simulink model "rou1_huibao_orthotropic_control"  (R2019b)
settings: Solver=ode23t  StartTime=0.0  StopTime=20  RelTol=1e-3
values from neighbouring files (symbols this model uses):
  I1 = 1    [HRGinitial.m]    (also in hrg_constr.m; untitled.m = 2000)
  I2 = 2500    [HRGinitial.m]    (also in hrg_constr.m; untitled.m = 1)
  I3 = 2000    [HRGinitial.m]    (also in hrg_constr.m = 2500; untitled.m = 2500)
  I4 = 2500    [HRGinitial.m]    (also in hrg_constr.m = 2000; untitled.m)
  K = 1.122    [HRGinitial.m]
  P1 = 0.2    [HRGinitial.m]    (also in hrg_constr.m; untitled.m = 40)
  P2 = 35    [HRGinitial.m]    (also in hrg_constr.m; untitled.m = 0.2)
  P3 = 40    [HRGinitial.m]    (also in hrg_constr.m = 35; untitled.m = 35)
  P4 = 35    [HRGinitial.m]    (also in hrg_constr.m = 40; untitled.m)
  x0 = [a*cos(omega*t+phi0)*cos(2*theta)-q*sin(omega*t+phi0)*sin(2*theta) ... (first row only)    [HRGinitial.m]
libraries: simulink x11, dsparch4 x4, dspswit3 x1, eeSinusoidalMeasurement x1, eeGeneralControl x1
settings Model: Creator=Administrator  LastModifiedBy=Administrator
settings SolverCC: AlgebraicLoopSolver=LineSearch

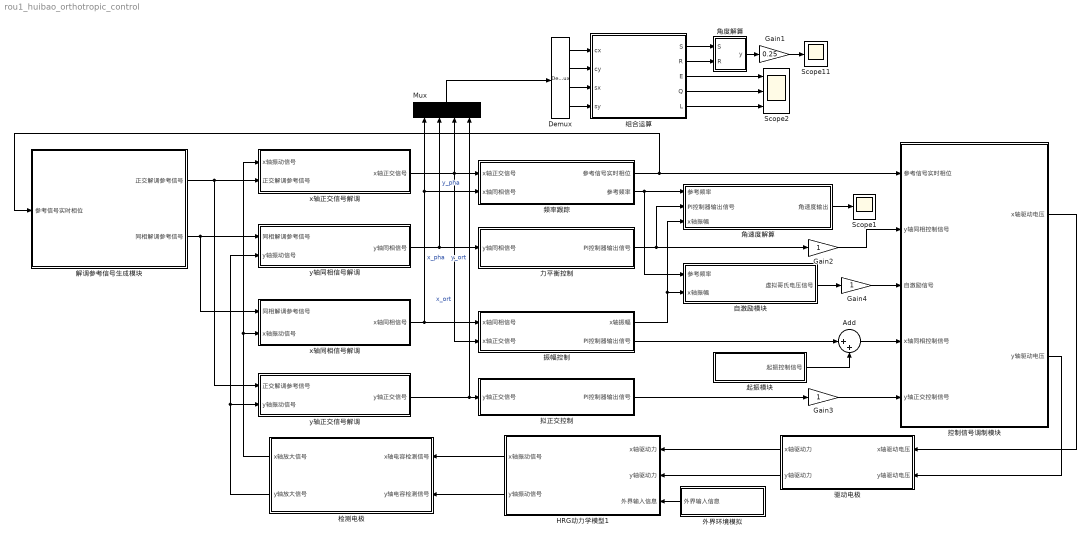
== system rou1_huibao_orthotropic_control ==
  Add : Sum  Inputs=|++
  Demux : Demux
  Gain1 : Gain  Gain=0.25
  Gain2 : Gain
  Gain3 : Gain
  Gain4 : Gain
  HRG动力学模型1 : Subsystem
  Mux : Mux
  Scope1 : Scope
  Scope11 : Scope
  Scope2 : Scope  NumInputPorts=3
  x轴同相信号解调 : Subsystem
  x轴正交信号解调 : Subsystem
  y轴同相信号解调 : Subsystem
  y轴正交信号解调 : Subsystem
  力平衡控制 : Subsystem
  外界环境模拟 : Subsystem
  拟正交控制 : Subsystem
  振幅控制 : Subsystem
  控制信号调制模块 : Subsystem
  检测电极 : Subsystem
  组合运算 : MATLAB Function  TreatAsAtomicUnit=on
  自激励模块 : Subsystem
  角度解算 : MATLAB Function  TreatAsAtomicUnit=on
  角速度解算 : Subsystem
  解调参考信号生成模块 : Subsystem
  起振模块 : Subsystem
  频率跟踪 : Subsystem
  驱动电极 : Subsystem
  wires:
  驱动电极/2(y轴驱动力) -> HRG动力学模型1/2(y轴驱动力)
  驱动电极/1(x轴驱动力) -> HRG动力学模型1/1(x轴驱动力)
  HRG动力学模型1/1(x轴振动信号) -> 检测电极/1(x轴电容检测信号)
  HRG动力学模型1/2(y轴振动信号) -> 检测电极/2(y轴电容检测信号)
  外界环境模拟/1(外界输入信息) -> HRG动力学模型1/3(外界输入信息)
  Demux/2 -> 组合运算/2(cy)
  组合运算/5(L) -> Scope2/3
  组合运算/3(E) -> Scope2/1
  解调参考信号生成模块/2(同相解调参考信号) -> y轴同相信号解调/1(同相解调参考信号), x轴同相信号解调/1(同相解调参考信号)
  Demux/3 -> 组合运算/3(sx)
  组合运算/2(R) -> 角度解算/2(R)
  自激励模块/1(虚拟哥氏电压信号) -> Gain4/1
  x轴同相信号解调/1(x轴同相信号) -> 振幅控制/1(x轴同相信号), 频率跟踪/2(x轴同相信号), Mux/1  "x_pha"
  Mux/1 -> Demux/1
  y轴同相信号解调/1(y轴同相信号) -> 力平衡控制/1(y轴同相信号), Mux/2  "y_pha"
  检测电极/2(y轴放大信号) -> y轴同相信号解调/2(y轴振动信号), y轴正交信号解调/2(y轴振动信号)
  控制信号调制模块/2(y轴驱动电压) -> 驱动电极/2(y轴驱动电压)
  组合运算/1(S) -> 角度解算/1(S)
  Gain1/1 -> Scope11/1
  检测电极/1(x轴放大信号) -> x轴正交信号解调/1(x轴振动信号), x轴同相信号解调/2(x轴振动信号)
  Add/1 -> 控制信号调制模块/4(x轴同相控制信号)
  振幅控制/1(x轴振幅) -> 角速度解算/3(x轴振幅), 自激励模块/2(x轴振幅)
  解调参考信号生成模块/1(正交解调参考信号) -> x轴正交信号解调/2(正交解调参考信号), y轴正交信号解调/1(正交解调参考信号)
  y轴正交信号解调/1(y轴正交信号) -> 拟正交控制/1(y轴正交信号), Mux/4  "y_ort"
  x轴正交信号解调/1(x轴正交信号) -> Mux/3, 频率跟踪/1(x轴正交信号), 振幅控制/2(x轴正交信号)  "x_ort"
  角速度解算/1(角速度输出) -> Scope1/1
  角度解算/1(y) -> Gain1/1
  组合运算/4(Q) -> Scope2/2
  频率跟踪/1(参考信号实时相位) -> 控制信号调制模块/1(参考信号实时相位), 解调参考信号生成模块/1(参考信号实时相位)
  控制信号调制模块/1(x轴驱动电压) -> 驱动电极/1(x轴驱动电压)
  起振模块/1(起振控制信号) -> Add/2
  力平衡控制/1(PI控制器输出信号) -> 角速度解算/2(PI控制器输出信号), Gain2/1
  Demux/1 -> 组合运算/1(cx)
  振幅控制/2(PI控制器输出信号) -> Add/1
  Demux/4 -> 组合运算/4(sy)
  频率跟踪/2(参考频率) -> 角速度解算/1(参考频率), 自激励模块/1(参考频率)
  拟正交控制/1(PI控制器输出信号) -> Gain3/1
  Gain2/1 -> 控制信号调制模块/2(y轴同相控制信号)
  Gain3/1 -> 控制信号调制模块/5(y轴正交控制信号)
  Gain4/1 -> 控制信号调制模块/3(自激励信号)

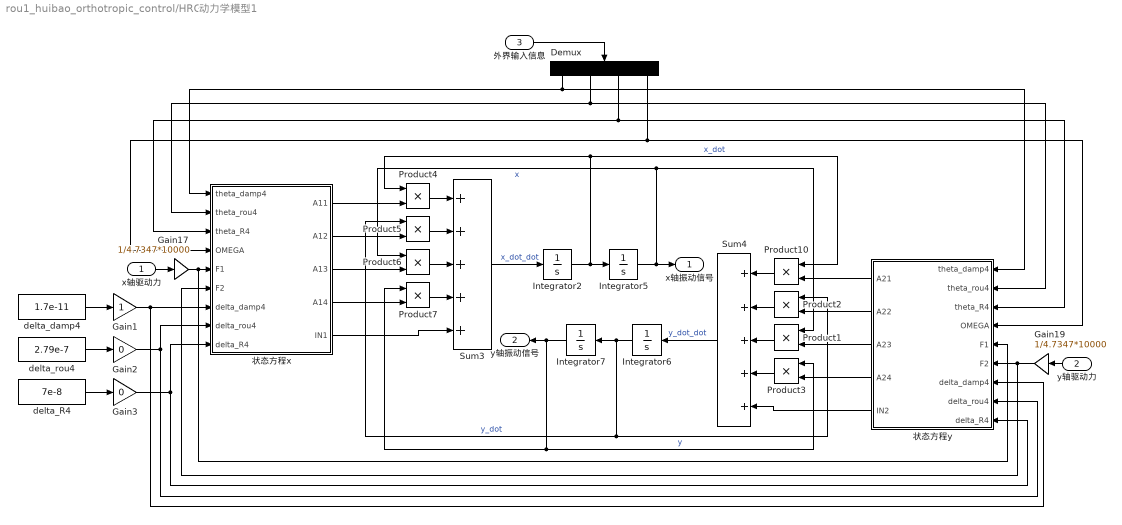
== system rou1_huibao_orthotropic_control/HRG动力学模型1 ==
  x轴驱动力 : Inport
  y轴驱动力 : Inport  Port=2
  外界输入信息 : Inport  Port=3
  Demux : Demux
  Gain1 : Gain
  Gain17 : Gain  Gain=1/4.7347*10000
  Gain19 : Gain  Gain=1/4.7347*10000
  Gain2 : Gain  Gain=0
  Gain3 : Gain  Gain=0
  Integrator2 : Integrator  InitialCondition=x0(3)
  Integrator5 : Integrator  InitialCondition=x0(1)
  Integrator6 : Integrator  InitialCondition=x0(4)
  Integrator7 : Integrator  InitialCondition=x0(2)
  Product{1..7,10} (8 alike) : Product
  Sum3 : Sum  Inputs=+++++
  Sum4 : Sum  Inputs=+++++
  delta_R4 : Constant  Value=7e-8
  delta_damp4 : Constant  Value=1.7e-11
  delta_rou4 : Constant  Value=2.79e-7
  状态方程x : MATLAB Function  TreatAsAtomicUnit=on
  状态方程y : MATLAB Function  TreatAsAtomicUnit=on
  x轴振动信号 : Outport
  y轴振动信号 : Outport  Port=2
  wires:
  y轴驱动力/1 -> Gain19/1
  x轴驱动力/1 -> Gain17/1
  Integrator2/1 -> Product4/1, Product10/1, Integrator5/1  "x_dot"
  Integrator6/1 -> Product2/1, Product5/1, Integrator7/1  "y_dot"
  Integrator7/1 -> Product3/1, Product7/1, y轴振动信号/1  "y"
  Sum3/1 -> Integrator2/1  "x_dot_dot"
  Integrator5/1 -> Product6/1, Product1/1, x轴振动信号/1  "x"
  Sum4/1 -> Integrator6/1  "y_dot_dot"
  状态方程x/5(IN1) -> Sum3/5
  Gain17/1 -> 状态方程y/5(F1), 状态方程x/5(F1)
  Gain19/1 -> 状态方程y/6(F2), 状态方程x/6(F2)
  Demux/1 -> 状态方程x/1(theta_damp4), 状态方程y/1(theta_damp4)
  Demux/2 -> 状态方程x/2(theta_rou4), 状态方程y/2(theta_rou4)
  Demux/3 -> 状态方程x/3(theta_R4), 状态方程y/3(theta_R4)
  Demux/4 -> 状态方程x/4(OMEGA), 状态方程y/4(OMEGA)
  外界输入信息/1 -> Demux/1
  状态方程y/5(IN2) -> Sum4/5
  Product1/1 -> Sum4/3
  Product2/1 -> Sum4/2
  Product10/1 -> Sum4/1
  Product3/1 -> Sum4/4
  Product4/1 -> Sum3/1
  Product5/1 -> Sum3/2
  Product6/1 -> Sum3/3
  Product7/1 -> Sum3/4
  状态方程x/1(A11) -> Product4/2
  状态方程x/2(A12) -> Product5/2
  状态方程x/3(A13) -> Product6/2
  状态方程x/4(A14) -> Product7/2
  状态方程y/1(A21) -> Product10/2
  状态方程y/2(A22) -> Product2/2
  状态方程y/3(A23) -> Product1/2
  状态方程y/4(A24) -> Product3/2
  delta_damp4/1 -> Gain1/1
  delta_R4/1 -> Gain3/1
  Gain1/1 -> 状态方程y/7(delta_damp4), 状态方程x/7(delta_damp4)
  delta_rou4/1 -> Gain2/1
  Gain2/1 -> 状态方程x/8(delta_rou4), 状态方程y/8(delta_rou4)
  Gain3/1 -> 状态方程y/9(delta_R4), 状态方程x/9(delta_R4)

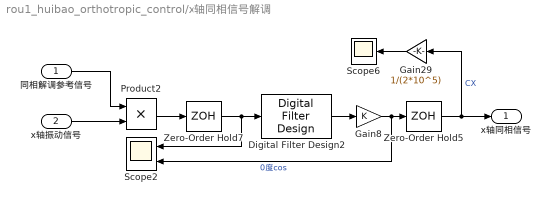
== system rou1_huibao_orthotropic_control/x轴同相信号解调 ==
  同相解调参考信号 : Inport
  x轴振动信号 : Inport  Port=2
  Digital Filter Design2 : dsparch4/Digital Filter Design  mwdsp_browser_bugfix_var=off
  Gain29 : Gain  Gain=1/(2*10^5)
  Gain8 : Gain  Gain=K
  Product2 : Product
  Scope2 : Scope  NumInputPorts=2
  Scope6 : Scope
  Zero-Order Hold5 : ZeroOrderHold  SampleTime=1/1000
  Zero-Order Hold7 : ZeroOrderHold  SampleTime=1/125000
  x轴同相信号 : Outport
  wires:
  Zero-Order Hold7/1 -> Scope2/1, Digital Filter Design2/1
  Zero-Order Hold5/1 -> Gain29/1, x轴同相信号/1  "CX"
  Product2/1 -> Zero-Order Hold7/1
  同相解调参考信号/1 -> Product2/1
  Gain8/1 -> Scope2/2, Zero-Order Hold5/1  "0度cos"
  Digital Filter Design2/1 -> Gain8/1
  x轴振动信号/1 -> Product2/2
  Gain29/1 -> Scope6/1

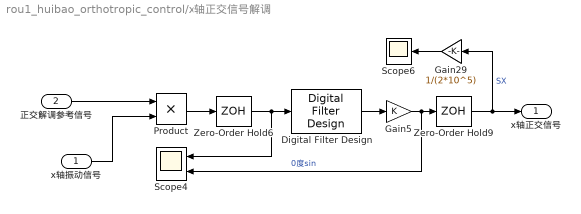
== system rou1_huibao_orthotropic_control/x轴正交信号解调 ==
  x轴振动信号 : Inport
  正交解调参考信号 : Inport  Port=2
  Digital Filter Design : dsparch4/Digital Filter Design  mwdsp_browser_bugfix_var=off
  Gain29 : Gain  Gain=1/(2*10^5)
  Gain5 : Gain  Gain=K
  Product : Product
  Scope4 : Scope  NumInputPorts=2
  Scope6 : Scope
  Zero-Order Hold6 : ZeroOrderHold  SampleTime=1/125000
  Zero-Order Hold9 : ZeroOrderHold  SampleTime=1/1000
  x轴正交信号 : Outport
  wires:
  Product/1 -> Zero-Order Hold6/1
  Zero-Order Hold9/1 -> Gain29/1, x轴正交信号/1  "SX"
  Gain5/1 -> Scope4/2, Zero-Order Hold9/1  "0度sin"
  Zero-Order Hold6/1 -> Scope4/1, Digital Filter Design/1
  x轴振动信号/1 -> Product/2
  Digital Filter Design/1 -> Gain5/1
  正交解调参考信号/1 -> Product/1
  Gain29/1 -> Scope6/1

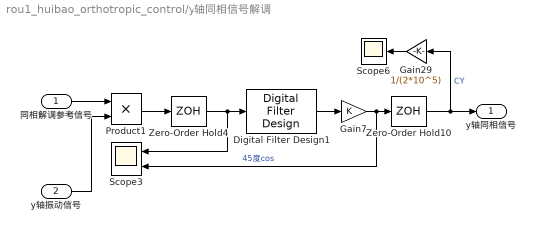
== system rou1_huibao_orthotropic_control/y轴同相信号解调 ==
  同相解调参考信号 : Inport
  y轴振动信号 : Inport  Port=2
  Digital Filter Design1 : dsparch4/Digital Filter Design  mwdsp_browser_bugfix_var=off
  Gain29 : Gain  Gain=1/(2*10^5)
  Gain7 : Gain  Gain=K
  Product1 : Product
  Scope3 : Scope  NumInputPorts=2
  Scope6 : Scope
  Zero-Order Hold10 : ZeroOrderHold  SampleTime=1/1000
  Zero-Order Hold4 : ZeroOrderHold  SampleTime=1/125000
  y轴同相信号 : Outport
  wires:
  Gain7/1 -> Scope3/2, Zero-Order Hold10/1  "45度cos"
  Digital Filter Design1/1 -> Gain7/1
  Zero-Order Hold4/1 -> Scope3/1, Digital Filter Design1/1
  y轴振动信号/1 -> Product1/2
  Zero-Order Hold10/1 -> Gain29/1, y轴同相信号/1  "CY"
  同相解调参考信号/1 -> Product1/1
  Product1/1 -> Zero-Order Hold4/1
  Gain29/1 -> Scope6/1

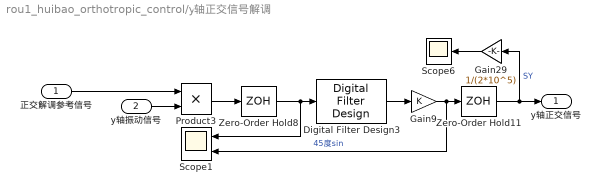
== system rou1_huibao_orthotropic_control/y轴正交信号解调 ==
  正交解调参考信号 : Inport
  y轴振动信号 : Inport  Port=2
  Digital Filter Design3 : dsparch4/Digital Filter Design  mwdsp_browser_bugfix_var=off
  Gain29 : Gain  Gain=1/(2*10^5)
  Gain9 : Gain  Gain=K
  Product3 : Product
  Scope1 : Scope  NumInputPorts=2
  Scope6 : Scope
  Zero-Order Hold11 : ZeroOrderHold  SampleTime=1/1000
  Zero-Order Hold8 : ZeroOrderHold  SampleTime=1/125000
  y轴正交信号 : Outport
  wires:
  Gain9/1 -> Scope1/2, Zero-Order Hold11/1  "45度sin"
  Product3/1 -> Zero-Order Hold8/1
  Zero-Order Hold8/1 -> Scope1/1, Digital Filter Design3/1
  Digital Filter Design3/1 -> Gain9/1
  正交解调参考信号/1 -> Product3/1
  y轴振动信号/1 -> Product3/2
  Zero-Order Hold11/1 -> Gain29/1, y轴正交信号/1  "SY"
  Gain29/1 -> Scope6/1

== system rou1_huibao_orthotropic_control/力平衡控制 ==
  y轴同相信号 : Inport
  Gain2 : Gain  Gain=-1
  Gain29 : Gain  Gain=1/(2*10^5)
  Gain33 : Gain  Gain=0.94694e5
  Scope5 : Scope
  Scope6 : Scope
  力平衡控制 : simulink/Continuous/PID Controller  Controller=PI  Form=Parallel  TimeDomain=Discrete-time  SampleTime=-1  IntegratorMethod=Forward Euler  FilterMethod=Forward Euler  ControllerParametersSource=internal  P=P4  I=I4  D=0  UseFilter=on  N=100  TunerSelectOption=Transfer Function Based (PID Tuner App)  InitialConditionSource=internal  InitialConditionForIntegrator=0  InitialConditionForFilter=0  DifferentiatorICPrevScaledInput=0  ExternalReset=none  TrackingMode=off  Kt=1  LimitOutput=off  UpperSaturationLimit=inf  LowerSaturationLimit=-inf  LinearizeAsGain=off  AntiWindupMode=none  Kb=1  POutMin=[]  POutMax=[]  IOutMin=[]  IOutMax=[]  DOutMin=[]  DOutMax=[]  NOutMin=[]  NOutMax=[]  SumOutMin=[]  SumOutMax=[]  SaturationOutMin=[]  SaturationOutMax=[]  PParamMin=[]  PParamMax=[]  IParamMin=[]  IParamMax=[]  DParamMin=[]  DParamMax=[]  NParamMin=[]  NParamMax=[]  KbParamMin=[]  KbParamMax=[]  KtParamMin=[]  KtParamMax=[]  KbOutMin=[]  KbOutMax=[]  KtOutMin=[]  KtOutMax=[]  IntegratorOutMin=[]  IntegratorOutMax=[]  FilterOutMin=[]  FilterOutMax=[]  SumI1OutMin=[]  SumI1OutMax=[]  SumI2OutMin=[]  SumI2OutMax=[]  SumI3OutMin=[]  SumI3OutMax=[]  SumI4OutMin=[]  SumI4OutMax=[]  SumDOutMin=[]  SumDOutMax=[]  DifferentiatorOutMin=[]  DifferentiatorOutMax=[]  FilterDiffOutCoefMin=[]  FilterDiffOutCoefMax=[]  ReciprocalOutMin=[]  ReciprocalOutMax=[]  SumDenOutMin=[]  SumDenOutMax=[]  SumNumOutMin=[]  SumNumOutMax=[]  DivideOutMin=[]  DivideOutMax=[]  IntegratorContinuousStateAttributes=''  IntegratorStateMustResolveToSignalObject=off  IntegratorRTWStateStorageClass=Auto  FilterContinuousStateAttributes=''  FilterStateMustResolveToSignalObject=off  FilterRTWStateStorageClass=Auto  ParallelPVariant=InternalParameters  IdealPVariant=Disabled  IVariant=InternalParameters  DVariant=Disabled  IntegratorVariant=Discrete  SatVariant=Disabled  AWVariant=Passthrough  PCopyVariant=Disabled  TRVariant=Disabled  FdbkBlocksVariant=Forward  IdealPFdbkVariant=Disabled  SatFdbkVariant=Disabled  DerivativeFilterVariant=Disabled  NVariant=Disabled  NCopyVariant=Disabled_SignalSpec  FilterICVariant=Disabled  IntegratorICVariant=InternalICs  ExternalResetVariant=Disabled  TRSumVariant=Passthrough  SumFdbkVariant=Disabled  SumVariant=Sum_PI
  PI控制器输出信号 : Outport
  wires:
  y轴同相信号/1 -> Gain2/1
  Gain29/1 -> Scope6/1
  Gain33/1 -> PI控制器输出信号/1
  Gain2/1 -> Gain29/1, 力平衡控制/1
  力平衡控制/1 -> Scope5/1, Gain33/1  "force_out"

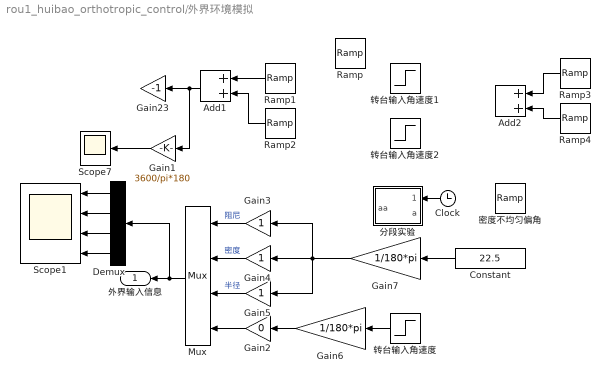
== system rou1_huibao_orthotropic_control/外界环境模拟 ==
  Add1 : Sum
  Add2 : Sum
  Clock : Clock
  Constant : Constant  Value=22.5  SampleTime=0
  Demux : Demux
  Gain1 : Gain  Gain=3600/pi*180
  Gain2 : Gain  Gain=0
  Gain23 : Gain  Gain=-1
  Gain3 : Gain
  Gain4 : Gain
  Gain5 : Gain
  Gain6 : Gain  Gain=1/180*pi
  Gain7 : Gain  Gain=1/180*pi
  Mux : Mux
  Ramp : simulink/Sources/Ramp  slope=7/3600/180*pi  start=7  InitialOutput=-45.5/3600/180*pi
  Ramp1 : simulink/Sources/Ramp  slope=100/180*pi  start=10  InitialOutput=0
  Ramp2 : simulink/Sources/Ramp  slope=-100/180*pi  start=10.1  InitialOutput=0
  Ramp3 : simulink/Sources/Ramp  slope=100/180*pi  start=0.3  InitialOutput=0
  Ramp4 : simulink/Sources/Ramp  slope=-100/180*pi  start=0.4  InitialOutput=0
  Scope1 : Scope  NumInputPorts=4
  Scope7 : Scope
  分段实验 : MATLAB Function  TreatAsAtomicUnit=on
  密度不均匀偏角 : simulink/Sources/Ramp  slope=2*pi/10  start=0  InitialOutput=0
  转台输入角速度 : Step  Time=10  After=20
  转台输入角速度1 : Step  Time=7  After=8.39446392/3600/180*pi
  转台输入角速度2 : Step  Time=6.5  Before=45.5/3600/180*pi  After=0
  外界输入信息 : Outport
  wires:
  Ramp2/1 -> Add1/2
  Ramp1/1 -> Add1/1
  Add1/1 -> Gain23/1, Gain1/1
  Gain1/1 -> Scope7/1
  Constant/1 -> Gain7/1
  Gain2/1 -> Mux/4
  Mux/1 -> Demux/1, 外界输入信息/1
  Ramp4/1 -> Add2/2
  Ramp3/1 -> Add2/1
  Demux/1 -> Scope1/1
  Demux/2 -> Scope1/2
  Demux/3 -> Scope1/3
  Demux/4 -> Scope1/4
  Gain3/1 -> Mux/1  "阻尼"
  Gain4/1 -> Mux/2  "密度"
  Gain5/1 -> Mux/3  "半径"
  Clock/1 -> 分段实验/1(clock)
  转台输入角速度/1 -> Gain6/1
  Gain7/1 -> Gain5/1, Gain4/1, Gain3/1
  Gain6/1 -> Gain2/1

== system rou1_huibao_orthotropic_control/拟正交控制 ==
  y轴正交信号 : Inport
  Gain1 : Gain  Gain=-1
  Gain28 : Gain  Gain=1/(2*10^5)
  Gain31 : Gain  Gain=0.94694e5
  Gain4 : Gain
  Scope8 : Scope
  Scope9 : Scope
  拟正交控制 : simulink/Continuous/PID Controller  Controller=PI  Form=Parallel  TimeDomain=Discrete-time  SampleTime=-1  IntegratorMethod=Forward Euler  FilterMethod=Forward Euler  ControllerParametersSource=internal  P=P2  I=I2  D=0  UseFilter=on  N=100  TunerSelectOption=Transfer Function Based (PID Tuner App)  InitialConditionSource=internal  InitialConditionForIntegrator=0  InitialConditionForFilter=0  DifferentiatorICPrevScaledInput=0  ExternalReset=none  TrackingMode=off  Kt=1  LimitOutput=off  UpperSaturationLimit=inf  LowerSaturationLimit=-inf  LinearizeAsGain=off  AntiWindupMode=none  Kb=1  POutMin=[]  POutMax=[]  IOutMin=[]  IOutMax=[]  DOutMin=[]  DOutMax=[]  NOutMin=[]  NOutMax=[]  SumOutMin=[]  SumOutMax=[]  SaturationOutMin=[]  SaturationOutMax=[]  PParamMin=[]  PParamMax=[]  IParamMin=[]  IParamMax=[]  DParamMin=[]  DParamMax=[]  NParamMin=[]  NParamMax=[]  KbParamMin=[]  KbParamMax=[]  KtParamMin=[]  KtParamMax=[]  KbOutMin=[]  KbOutMax=[]  KtOutMin=[]  KtOutMax=[]  IntegratorOutMin=[]  IntegratorOutMax=[]  FilterOutMin=[]  FilterOutMax=[]  SumI1OutMin=[]  SumI1OutMax=[]  SumI2OutMin=[]  SumI2OutMax=[]  SumI3OutMin=[]  SumI3OutMax=[]  SumI4OutMin=[]  SumI4OutMax=[]  SumDOutMin=[]  SumDOutMax=[]  DifferentiatorOutMin=[]  DifferentiatorOutMax=[]  FilterDiffOutCoefMin=[]  FilterDiffOutCoefMax=[]  ReciprocalOutMin=[]  ReciprocalOutMax=[]  SumDenOutMin=[]  SumDenOutMax=[]  SumNumOutMin=[]  SumNumOutMax=[]  DivideOutMin=[]  DivideOutMax=[]  IntegratorContinuousStateAttributes=''  IntegratorStateMustResolveToSignalObject=off  IntegratorRTWStateStorageClass=Auto  FilterContinuousStateAttributes=''  FilterStateMustResolveToSignalObject=off  FilterRTWStateStorageClass=Auto  ParallelPVariant=InternalParameters  IdealPVariant=Disabled  IVariant=InternalParameters  DVariant=Disabled  IntegratorVariant=Discrete  SatVariant=Disabled  AWVariant=Passthrough  PCopyVariant=Disabled  TRVariant=Disabled  FdbkBlocksVariant=Forward  IdealPFdbkVariant=Disabled  SatFdbkVariant=Disabled  DerivativeFilterVariant=Disabled  NVariant=Disabled  NCopyVariant=Disabled_SignalSpec  FilterICVariant=Disabled  IntegratorICVariant=InternalICs  ExternalResetVariant=Disabled  TRSumVariant=Passthrough  SumFdbkVariant=Disabled  SumVariant=Sum_PI
  正交控制力是否为0 : Subsystem
  PI控制器输出信号 : Outport
  wires:
  y轴正交信号/1 -> Gain1/1
  Gain31/1 -> Scope8/1, 正交控制力是否为0/1(In1), Gain4/1
  Gain4/1 -> PI控制器输出信号/1
  Gain1/1 -> 拟正交控制/1, Gain28/1
  拟正交控制/1 -> Gain31/1  "Quasi_orthogonal"
  Gain28/1 -> Scope9/1

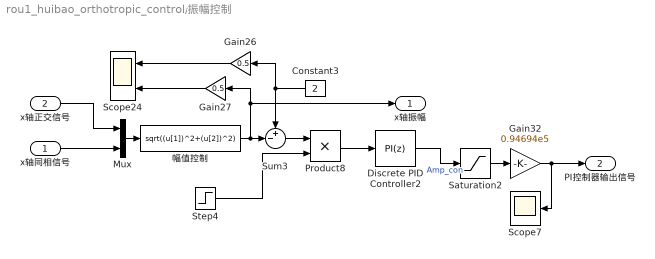
== system rou1_huibao_orthotropic_control/振幅控制 ==
  x轴同相信号 : Inport
  x轴正交信号 : Inport  Port=2
  Constant3 : Constant  Value=2  SampleTime=1/1000
  Discrete PID Controller2 : simulink/Continuous/PID Controller  Controller=PI  Form=Parallel  TimeDomain=Discrete-time  SampleTime=-1  IntegratorMethod=Forward Euler  FilterMethod=Forward Euler  ControllerParametersSource=internal  P=P1  I=I1  D=0  UseFilter=on  N=100  TunerSelectOption=Transfer Function Based (PID Tuner App)  InitialConditionSource=internal  InitialConditionForIntegrator=0  InitialConditionForFilter=0  DifferentiatorICPrevScaledInput=0  ExternalReset=none  TrackingMode=off  Kt=1  LimitOutput=off  UpperSaturationLimit=inf  LowerSaturationLimit=-inf  LinearizeAsGain=off  AntiWindupMode=none  Kb=1  POutMin=[]  POutMax=[]  IOutMin=[]  IOutMax=[]  DOutMin=[]  DOutMax=[]  NOutMin=[]  NOutMax=[]  SumOutMin=[]  SumOutMax=[]  SaturationOutMin=[]  SaturationOutMax=[]  PParamMin=[]  PParamMax=[]  IParamMin=[]  IParamMax=[]  DParamMin=[]  DParamMax=[]  NParamMin=[]  NParamMax=[]  KbParamMin=[]  KbParamMax=[]  KtParamMin=[]  KtParamMax=[]  KbOutMin=[]  KbOutMax=[]  KtOutMin=[]  KtOutMax=[]  IntegratorOutMin=[]  IntegratorOutMax=[]  FilterOutMin=[]  FilterOutMax=[]  SumI1OutMin=[]  SumI1OutMax=[]  SumI2OutMin=[]  SumI2OutMax=[]  SumI3OutMin=[]  SumI3OutMax=[]  SumI4OutMin=[]  SumI4OutMax=[]  SumDOutMin=[]  SumDOutMax=[]  DifferentiatorOutMin=[]  DifferentiatorOutMax=[]  FilterDiffOutCoefMin=[]  FilterDiffOutCoefMax=[]  ReciprocalOutMin=[]  ReciprocalOutMax=[]  SumDenOutMin=[]  SumDenOutMax=[]  SumNumOutMin=[]  SumNumOutMax=[]  DivideOutMin=[]  DivideOutMax=[]  IntegratorContinuousStateAttributes=''  IntegratorStateMustResolveToSignalObject=off  IntegratorRTWStateStorageClass=Auto  FilterContinuousStateAttributes=''  FilterStateMustResolveToSignalObject=off  FilterRTWStateStorageClass=Auto  ParallelPVariant=InternalParameters  IdealPVariant=Disabled  IVariant=InternalParameters  DVariant=Disabled  IntegratorVariant=Discrete  SatVariant=Disabled  AWVariant=Passthrough  PCopyVariant=Disabled  TRVariant=Disabled  FdbkBlocksVariant=Forward  IdealPFdbkVariant=Disabled  SatFdbkVariant=Disabled  DerivativeFilterVariant=Disabled  NVariant=Disabled  NCopyVariant=Disabled_SignalSpec  FilterICVariant=Disabled  IntegratorICVariant=InternalICs  ExternalResetVariant=Disabled  TRSumVariant=Passthrough  SumFdbkVariant=Disabled  SumVariant=Sum_PI
  Gain26 : Gain  Gain=0.5
  Gain27 : Gain  Gain=0.5
  Gain32 : Gain  Gain=0.94694e5
  Mux : Mux  Inputs=2
  Product8 : Product
  Saturation2 : Saturate  UpperLimit=2e7  LowerLimit=-2e7
  Scope24 : Scope  NumInputPorts=2
  Scope7 : Scope
  Step4 : Step  Time=5.98  SampleTime=1/1000
  Sum3 : Sum  Inputs=+-|
  幅值控制 : Fcn  Expr=sqrt((u[1])^2+(u[2])^2)
  x轴振幅 : Outport
  PI控制器输出信号 : Outport  Port=2
  wires:
  幅值控制/1 -> x轴振幅/1, Gain27/1, Sum3/2
  Constant3/1 -> Sum3/1, Gain26/1
  Gain26/1 -> Scope24/1
  Gain27/1 -> Scope24/2
  Gain32/1 -> PI控制器输出信号/1, Scope7/1
  Discrete PID Controller2/1 -> Saturation2/1  "Amp_con"
  x轴同相信号/1 -> Mux/2
  Mux/1 -> 幅值控制/1
  Saturation2/1 -> Gain32/1
  x轴正交信号/1 -> Mux/1
  Sum3/1 -> Product8/1
  Step4/1 -> Product8/2
  Product8/1 -> Discrete PID Controller2/1

== system rou1_huibao_orthotropic_control/控制信号调制模块 ==
  参考信号实时相位 : Inport
  y轴同相控制信号 : Inport  Port=2
  自激励信号 : Inport  Port=3
  x轴同相控制信号 : Inport  Port=4
  y轴正交控制信号 : Inport  Port=5
  控制信号调制模块 : MATLAB Function  TreatAsAtomicUnit=on
  x轴驱动电压 : Outport
  y轴驱动电压 : Outport  Port=2
  wires:
  x轴同相控制信号/1 -> 控制信号调制模块/4(Fx)
  y轴正交控制信号/1 -> 控制信号调制模块/5(Fy2)
  控制信号调制模块/2(VY) -> y轴驱动电压/1
  控制信号调制模块/1(VX) -> x轴驱动电压/1
  y轴同相控制信号/1 -> 控制信号调制模块/2(Fy1)
  参考信号实时相位/1 -> 控制信号调制模块/1(fai1)
  自激励信号/1 -> 控制信号调制模块/3(selfcal)

== system rou1_huibao_orthotropic_control/检测电极 ==
  x轴电容检测信号 : Inport
  y轴电容检测信号 : Inport  Port=2
  Add : Sum
  Add1 : Sum
  Gain1 : Gain  Gain=2*10^5
  Gain35 : Gain  Gain=2*10^5
  Random Number : RandomNumber  Variance=0.0001  SampleTime=1e-6
  Scope1 : Scope  NumInputPorts=2
  Scope2 : Scope  NumInputPorts=2
  x轴放大信号 : Outport
  y轴放大信号 : Outport  Port=2
  wires:
  Add1/1 -> Scope1/2, y轴放大信号/1
  x轴电容检测信号/1 -> Scope2/1, Gain35/1
  y轴电容检测信号/1 -> Scope2/2, Gain1/1
  Add/1 -> Scope1/1, x轴放大信号/1
  Gain35/1 -> Add/1
  Gain1/1 -> Add1/2

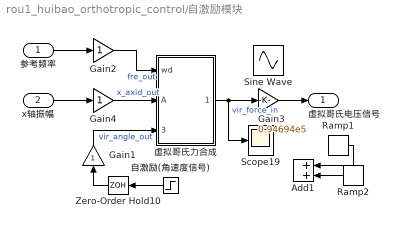
== system rou1_huibao_orthotropic_control/自激励模块 ==
  参考频率 : Inport
  x轴振幅 : Inport  Port=2
  Add1 : Sum
  Gain1 : Gain
  Gain2 : Gain
  Gain3 : Gain  Gain=0.94694e5
  Gain4 : Gain
  Ramp1 : simulink/Sources/Ramp  slope=100/180*pi  start=0.3  InitialOutput=0
  Ramp2 : simulink/Sources/Ramp  slope=-100/180*pi  start=0.4  InitialOutput=0
  Scope19 : Scope
  Sine Wave : Sin  SampleTime=0
  Zero-Order Hold10 : ZeroOrderHold  SampleTime=1/1000
  自激励(角速度信号) : Step  Time=10  After=10  SampleTime=1/1000
  虚拟哥氏力合成 : MATLAB Function  TreatAsAtomicUnit=on
  虚拟哥氏电压信号 : Outport
  wires:
  虚拟哥氏力合成/1(output) -> Scope19/1, Gain3/1  "vir_force_in"
  Gain1/1 -> 虚拟哥氏力合成/3(OMEGA)  "vir_angle_out"
  Ramp2/1 -> Add1/2
  Ramp1/1 -> Add1/1
  Zero-Order Hold10/1 -> Gain1/1
  Gain2/1 -> 虚拟哥氏力合成/1(wd)  "fre_out"
  Gain4/1 -> 虚拟哥氏力合成/2(A)  "x_axid_out"
  参考频率/1 -> Gain2/1
  x轴振幅/1 -> Gain4/1
  Gain3/1 -> 虚拟哥氏电压信号/1
  自激励(角速度信号)/1 -> Zero-Order Hold10/1

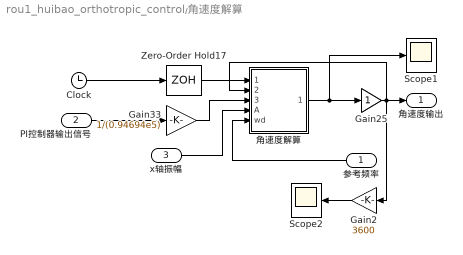
== system rou1_huibao_orthotropic_control/角速度解算 ==
  参考频率 : Inport
  PI控制器输出信号 : Inport  Port=2
  x轴振幅 : Inport  Port=3
  Clock : Clock
  Gain2 : Gain  Gain=3600
  Gain25 : Gain
  Gain33 : Gain  Gain=1/(0.94694e5)
  Scope1 : Scope
  Scope2 : Scope
  Zero-Order Hold17 : ZeroOrderHold  SampleTime=1/1000
  角速度解算 : MATLAB Function  TreatAsAtomicUnit=on
  角速度输出 : Outport
  wires:
  参考频率/1 -> 角速度解算/5(wd)
  Zero-Order Hold17/1 -> 角速度解算/1(clock)
  Clock/1 -> Zero-Order Hold17/1
  角速度解算/1(OMEGA) -> Scope1/1, Gain25/1
  Gain25/1 -> 角速度解算/2(OMEGA1), Gain2/1, 角速度输出/1
  x轴振幅/1 -> 角速度解算/4(A)
  Gain33/1 -> 角速度解算/3(output)
  Gain2/1 -> Scope2/1
  PI控制器输出信号/1 -> Gain33/1

== system rou1_huibao_orthotropic_control/解调参考信号生成模块 ==
  参考信号实时相位 : Inport
  sin : Fcn  Expr=2*cos(u[1])
  sin1 : Fcn  Expr=2*sin(u[1])
  正交解调参考信号 : Outport
  同相解调参考信号 : Outport  Port=2
  wires:
  参考信号实时相位/1 -> sin1/1, sin/1
  sin/1 -> 同相解调参考信号/1
  sin1/1 -> 正交解调参考信号/1

== system rou1_huibao_orthotropic_control/起振模块 ==
  Gain : Gain
  起振控制1信号 : Step  Time=5.98  Before=10000  After=0  SampleTime=1/1000
  起振控制信号 : Outport
  wires:
  起振控制1信号/1 -> Gain/1
  Gain/1 -> 起振控制信号/1

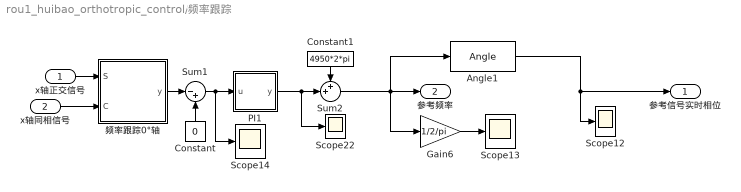
== system rou1_huibao_orthotropic_control/频率跟踪 ==
  x轴正交信号 : Inport
  x轴同相信号 : Inport  Port=2
  Angle1 : eeSinusoidalMeasurement/Sinusoidal Measurement (PLL)/Angle  SystemSampleTime=-1  Latency=0  AutoFrameSizeCalculation=off
      link override Integrator with Wrapped State (Discrete or Continuous): x0=0  Ts=1e-6
      settings: SourceProductName=Simscape Electrical  SourceProductBaseCode=PS
  Constant : Constant  Value=0
  Constant1 : Constant  Value=4950*2*pi
  Gain6 : Gain  Gain=1/2/pi
  PI1 : Subsystem  AncestorBlock=|
      | eeSinusoidalMeasurement/Sinusoidal Measurement
      | (PLL)/PI
  Scope{12..14,22} (4 alike) : Scope
  Sum1 : Sum  Inputs=|-+
  Sum2 : Sum  Inputs=++|
  频率跟踪0°轴 : MATLAB Function  TreatAsAtomicUnit=on
  参考信号实时相位 : Outport
  参考频率 : Outport  Port=2
  wires:
  x轴同相信号/1 -> 频率跟踪0°轴/2(C)
  PI1/1(y) -> Sum2/2, Scope22/1
  Constant/1 -> Sum1/2
  Gain6/1 -> Scope13/1
  Constant1/1 -> Sum2/1
  Sum1/1 -> PI1/1(u), Scope14/1
  频率跟踪0°轴/1(y) -> Sum1/1
  Angle1/1 -> Scope12/1, 参考信号实时相位/1
  Sum2/1 -> Gain6/1, Angle1/1, 参考频率/1
  x轴正交信号/1 -> 频率跟踪0°轴/1(S)

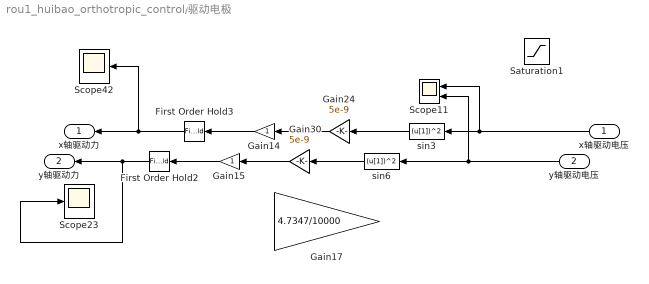
== system rou1_huibao_orthotropic_control/驱动电极 ==
  x轴驱动电压 : Inport
  y轴驱动电压 : Inport  Port=2
  First Order Hold2 : FirstOrderHold  ErrorTolerance=inf
  First Order Hold3 : FirstOrderHold  ErrorTolerance=inf
  Gain14 : Gain
  Gain15 : Gain
  Gain17 : Gain  Gain=4.7347/10000
  Gain24 : Gain  Gain=5e-9
  Gain30 : Gain  Gain=5e-9
  Saturation1 : Saturate  UpperLimit=200  LowerLimit=-200
  Scope11 : Scope  NumInputPorts=2
  Scope23 : Scope
  Scope42 : Scope
  sin3 : Fcn  Expr=(u[1])^2
  sin6 : Fcn  Expr=(u[1])^2
  x轴驱动力 : Outport
  y轴驱动力 : Outport  Port=2
  wires:
  Gain14/1 -> First Order Hold3/1
  x轴驱动电压/1 -> sin3/1, Scope11/1
  sin6/1 -> Gain30/1
  y轴驱动电压/1 -> sin6/1, Scope11/2
  Gain15/1 -> First Order Hold2/1
  Gain24/1 -> Gain14/1
  Gain30/1 -> Gain15/1
  sin3/1 -> Gain24/1
  First Order Hold2/1 -> Scope23/1, y轴驱动力/1
  First Order Hold3/1 -> Scope42/1, x轴驱动力/1

== system rou1_huibao_orthotropic_control/拟正交控制/正交控制力是否为0 ==
  In1 : Inport
  Counter1 : dspswit3/Counter  Direction=Up  CountEvent=Rising edge  CounterSize=User defined  MaxCount=1e10  InitialCount=0  Output=Count  HitValue=32  ResetInput=off  SamplesPerFrame=1  Ts=1  CntDtype=double  HitDtype=Logical
  Pulse Generator1 : DiscretePulseGenerator  PulseType=Time based  Period=1/1000  PulseWidth=50
  Scope : Scope
  Scope1 : Scope
  Scope2 : Scope
  Step1 : Step  Time=0  After=0  SampleTime=1/1000/2
  Switch1 : Switch  Criteria=u2 ~= 0  Threshold=1000
  Zero-Order Hold1 : ZeroOrderHold  SampleTime=1/1000/2
  wires:
  In1/1 -> Zero-Order Hold1/1, Scope/1
  Counter1/1 -> Scope2/1
  Pulse Generator1/1 -> Switch1/3
  Step1/1 -> Switch1/1
  Switch1/1 -> Counter1/1, Scope1/1
  Zero-Order Hold1/1 -> Switch1/2

== system rou1_huibao_orthotropic_control/频率跟踪/PI1 ==
  u : Inport
  Constant : Constant  Value=0
  Constant1 : Constant  Value=0
  Gain : Gain  Gain=P3
  Gain1 : Gain  Gain=I3
  Integrator (Discrete or Continuous) : eeGeneralControl/Integrator (Discrete or Continuous)  LabelModeActiveChoice=Discrete  ExternalReset=level  LimitType=Anti-windup  B=inf  A=-inf  Ts=-1
      settings: SourceProductName=Simscape Electrical  SourceProductBaseCode=PS
  Sum : Sum  Inputs=|++
  y : Outport  VectorParamsAs1DForOutWhenUnconnected=off
  wires:
  Constant1/1 -> Integrator (Discrete or Continuous)/2
  Constant/1 -> Integrator (Discrete or Continuous)/3
  Sum/1 -> y/1
  Integrator (Discrete or Continuous)/1 -> Sum/2
  Gain/1 -> Sum/1
  u/1 -> Gain/1, Gain1/1
  Gain1/1 -> Integrator (Discrete or Continuous)/1

== matlab function rou1_huibao_orthotropic_control/HRG动力学模型1/状态方程x ==
  data: theta_damp4 input; theta_rou4 input; theta_R4 input; OMEGA input; A11 output; A12 output; A13 output; A14 output; IN1 output; F1 input; F2 input; delta_damp4 input; delta_rou4 input; delta_R4 input
function [A11,A12,A13,A14,IN1] = state_eq(theta_damp4,theta_rou4,...
    theta_R4,OMEGA,F1,F2,delta_damp4,delta_rou4,delta_R4)
%% 仿真参数
m0=1.52961; m1=0.55296; b0=-0.42369; e0=1.05922; e1=0.31777;
omega = 4964.703945*2*pi; k = 0.277; %固有频率和进动因子
E=7.76e10; gamma=0.17; h=0.85e-3; %杨氏模量、泊松比和厚度
azi_theta=0; %角速度输入值和驻波方位角
Q=5e6; %品质因数平均值
%% 阻尼不均匀
ava_damp_x=0.0015188;
ava_damp=0.0031194;
a_damp4=delta_damp4*cos(4*theta_damp4);
b_damp4=delta_damp4*sin(4*theta_damp4);
%% 密度不均匀
ava_rou=2200;
a_rou4=delta_rou4*cos(4*theta_rou4);
b_rou4=delta_rou4*sin(4*theta_rou4);
%% 半径不均匀
ava_R=0.015;
a_R4=delta_R4*cos(4*theta_R4);
b_R4=delta_R4*sin(4*theta_R4);
%% 状态方程构建
A11=1/(-(m0+m1*a_rou4)*(m0-m1*a_rou4)+(m1*b_rou4)^2)*...
    ((m0-m1*a_rou4)*ava_damp_x*(1+m1*a_damp4/m0-4*m1*a_R4/m0)-...
    m1*b_rou4*(-4*OMEGA*b0+ava_damp_x*(m1*b_damp4/m0-4*m1*b_R4/m0)));
A12=1/(-(m0+m1*a_rou4)*(m0-m1*a_rou4)+(m1*b_rou4)^2)*...
    ((m0-m1*a_rou4)*(4*OMEGA*b0+ava_damp_x*(m1*b_damp4/m0-4*m1*b_R4/m0))-...
    m1*b_rou4*ava_damp_x*(1-m1*a_damp4/m0+4*m1*a_R4/m0));
A13=1/(-(m0+m1*a_rou4)*(m0-m1*a_rou4)+(m1*b_rou4)^2)*...
    ((m0-m1*a_rou4)*((m0-4*m1*a_R4)*omega^2-(e0+e1*a_rou4)*OMEGA^2)-...
    m1*b_rou4*(-4*m1*b_R4*omega^2-e1*b_rou4*OMEGA^2));
A14=1/(-(m0+m1*a_rou4)*(m0-m1*a_rou4)+(m1*b_rou4)^2)*...
    ((m0-m1*a_rou4)*(-4*m1*b_R4*omega^2-e1*b_rou4*OMEGA^2)-...
    m1*b_rou4*((m0+4*m1*a_R4)*omega^2-(e0-e1*a_rou4)*OMEGA^2));
B11=1/(-(m0+m1*a_rou4)*(m0-m1*a_rou4)+(m1*b_rou4)^2)*(-1)*(m0-m1*a_rou4)*(m0+m1*a_rou4);
B12=1/(-(m0+m1*a_rou4)*(m0-m1*a_rou4)+(m1*b_rou4)^2)*m1*b_rou4*(m0-m1*a_rou4);
IN1=(B11*F1+B12*F2);

== matlab function rou1_huibao_orthotropic_control/HRG动力学模型1/状态方程y ==
  data: theta_damp4 input; theta_rou4 input; theta_R4 input; OMEGA input; A21 output; A22 output; A23 output; A24 output; IN2 output; F1 input; F2 input; delta_damp4 input; delta_rou4 input; delta_R4 input
function [A21,A22,A23,A24,IN2] = state_eq(theta_damp4,theta_rou4,...
    theta_R4,OMEGA,F1,F2,delta_damp4,delta_rou4,delta_R4)
%% 仿真参数
m0=1.52961; m1=0.55296; b0=-0.42369; e0=1.05922; e1=0.31777;
omega = 4964.703945*2*pi; k = 0.277; %固有频率和进动因子
E=7.76e10; gamma=0.17; h=0.85e-3; %杨氏模量、泊松比和厚度
azi_theta=0; %角速度输入值和驻波方位角
Q=5e6; %品质因数平均值
%% 阻尼不均匀
ava_damp_x=0.0015188;
ava_damp=0.0031194;
a_damp4=delta_damp4*cos(4*theta_damp4);
b_damp4=delta_damp4*sin(4*theta_damp4);
%% 密度不均匀
ava_rou=2200;
a_rou4=delta_rou4*cos(4*theta_rou4);
b_rou4=delta_rou4*sin(4*theta_rou4);
%% 半径不均匀
ava_R=0.015;
a_R4=delta_R4*cos(4*theta_R4);
b_R4=delta_R4*sin(4*theta_R4);
%% 状态方程构建
A21=1/(-(m1*b_rou4)^2+(m0+m1*a_rou4)*(m0-m1*a_rou4))*...
    (m1*b_rou4*ava_damp_x*(1+m1*a_damp4/m0-4*m1*a_R4/m0)-...
    (m0+m1*a_rou4)*(-4*OMEGA*b0+ava_damp_x*(m1*b_damp4/m0-4*m1*b_R4/m0)));
A22=1/(-(m1*b_rou4)^2+(m0+m1*a_rou4)*(m0-m1*a_rou4))*...
    (m1*b_rou4*(4*OMEGA*b0+ava_damp_x*(m1*b_damp4/m0-4*m1*b_R4/m0))-...
    (m0+m1*a_rou4)*ava_damp_x*(1-m1*a_damp4/m0+4*m1*a_R4/m0));
A23=1/(-(m1*b_rou4)^2+(m0+m1*a_rou4)*(m0-m1*a_rou4))*...
    (m1*b_rou4*((m0-4*m1*a_R4)*omega^2-(e0+e1*a_rou4)*OMEGA^2)-...
    (m0+m1*a_rou4)*(-4*m1*b_R4*omega^2-e1*b_rou4*OMEGA^2));
A24=1/(-(m1*b_rou4)^2+(m0+m1*a_rou4)*(m0-m1*a_rou4))*...
    (m1*b_rou4*(-4*m1*b_R4*omega^2-e1*b_rou4*OMEGA^2)-...
    (m0+m1*a_rou4)*((m0+4*m1*a_R4)*omega^2-(e0-e1*a_rou4)*OMEGA^2));
B21=1/(-(m1*b_rou4)^2+(m0+m1*a_rou4)*(m0-m1*a_rou4))*(-1)*m1*b_rou4*(m0+m1*a_rou4);
B22=1/(-(m1*b_rou4)^2+(m0+m1*a_rou4)*(m0-m1*a_rou4))*(m0+m1*a_rou4)*(m0-m1*a_rou4);
IN2=(B21*F1+B22*F2);

== matlab function rou1_huibao_orthotropic_control/组合运算 ==
  data: S output; R output; cx input; E output; cy input; sx input; sy input; Q output; L output
function [S,R,E,Q,L] = zuheyunsuan(cx,cy,sx,sy)
E = cx^2+cy^2+sx^2+sy^2;
Q=2*(cx*sy-cy*sx);
S=2*(cx*cy+sy*sx);
R=cx^2-cy^2+sx^2-sy^2;
L=2*(cx*sx+cy*sy);

== matlab function rou1_huibao_orthotropic_control/控制信号调制模块/控制信号调制模块 ==
  data: fai1 input; Fy1 input; selfcal input; Fx input; VX output; VY output; Fy2 input
function [VX,VY] = qdhcytz(fai1,Fy1,selfcal,Fx,Fy2)
y1=0;y2=0;
if Fy2 ~= 0
    if (Fy1-selfcal) >= 0
        if Fy2 > 0
            y1 = atan((Fy1-selfcal)/Fy2);
        else
            y1 = (pi + atan((Fy1-selfcal)/Fy2) );
        end
    else
        if Fy2 > 0
            y1 = ( atan((Fy1-selfcal)/Fy2) );
        else
            y1 = ( atan((Fy1-selfcal)/Fy2) - pi);
        end
    end
end

if Fy2 ~= 0
    if (Fy1-selfcal) >= 0
        if (-Fy2) > 0
            y2 = atan((Fy1-selfcal)/-Fy2);
        else
            y2 = (pi + atan((Fy1-selfcal)/-Fy2) );
        end
    else
        if (-Fy2) > 0
            y2 = ( atan((Fy1-selfcal)/-Fy2) );
        else
            y2 = ( atan((Fy1-selfcal)/-Fy2) - pi);
        end
    end
end

if Fx < 0
    VX = sqrt(-2*Fx)*sin(fai1/2 + pi/4);
else
    VX = sqrt(2*Fx)*cos(fai1/2 + pi/4);
end
if Fy2 < 0
    VY = sqrt(2*sqrt((Fy1-selfcal)^2+Fy2^2))*sin(fai1/2-0.5*y2);
else
    VY = sqrt(2*sqrt((Fy1-selfcal)^2+Fy2^2))*cos(fai1/2+0.5*y1);
end

== matlab function rou1_huibao_orthotropic_control/角度解算 ==
  data: S input; y output; R input
function y = jdjs(S,R)
y = 0;
if R ~= 0
    if S >= 0
        if R > 0
            y = atan(S/R);
        else
            y = (pi + atan(S/R) );
        end
    else
        if R > 0
            y = ( atan(S/R) );
        else
            y = ( atan(S/R) - pi);
        end
    end
end

== matlab function rou1_huibao_orthotropic_control/自激励模块/虚拟哥氏力合成 ==
  data: wd input; A input; OMEGA input; output output
function output  = coriolis_vir(wd,A,OMEGA)
m0=1.52961; m1=0.55296; b0=-0.42369; e0=1.05922; e1=0.31777;
output=4*(-b0/m0)*OMEGA/180*pi*A/2e5*wd;

== matlab function rou1_huibao_orthotropic_control/角速度解算/角速度解算 ==
  data: clock input; OMEGA1 input; output input; A input; wd input; OMEGA output
function OMEGA  = coriolis_vir(clock,OMEGA1,output,A,wd)
m0=1.52961; m1=0.55296; b0=-0.42369; e0=1.05922; e1=0.31777;
if clock<=1/200
    OMEGA=0;
else
    OMEGA=OMEGA1;
end
if A ~=0
    OMEGA=output/(4*(-b0/m0)*A/200000*wd)/pi*180;
end

== matlab function rou1_huibao_orthotropic_control/频率跟踪/频率跟踪0°轴 ==
  data: S input; C input; y output
function y = jdjs(S,C)
y = 0;
if C ~= 0
    if S >= 0
        if C > 0
            y = atan(S/C);
        else
            y = (pi + atan(S/C) );
        end
    else
        if C > 0
            y = ( atan(S/C) );
        else
            y = ( atan(S/C) - pi);
        end
    end
end

== matlab function rou1_huibao_orthotropic_control/外界环境模拟/分段实验 ==
  data: clock input; a input; aa output
function aa = timedis(clock,a)
aa=0;
if clock>0   %1
    aa=a*0;
end
if clock>5.5   %2
    aa=a*1;
end
if clock>11    %3
    aa=a*2;
end
if clock>16.5     %4
    aa=a*3;
end
if clock>22.5    %5
    aa=a*4;
end
if clock>27.5    %6
    aa=a*5;
end
if clock>33    %7
    aa=a*6;
end
if clock>38.5    %8
    aa=a*7;
end
if clock>44    %9
    aa=a*8;
end
if clock>49.5    %10
    aa=a*9;
end
